simulink model "main"  (R2021a)
settings: Solver=ode45  StartTime=50  StopTime=60  RelTol=1e-3  EnableMultiTasking=on
undefined symbols (not defined in the file): Cadmium, Nickel
libraries: spsSeriesRLCBranchLib x4, spsGroundLib x3, spsControlledVoltageSourceLib x3, spsCurrentMeasurementLib x2, spsVoltageMeasurementLib x2, spspowerguiLib x2, spsBatteryLib x1, spsDiodeLib x1, spsMosfetLib x1, spsPWMGeneratorDCDCLib x1, spsUniversalBridgeLib x1
settings Model: Creator=Waqas vicky  LastModifiedBy=Le General
settings SolverCC: AlgebraicLoopSolver=TrustRegion
settings DataIOCC: LimitDataPoints=on  SaveFormat=Array  SignalLoggingSaveFormat=ModelDataLogs  ReturnWorkspaceOutputs=off
settings OptimizationCC: ExpressionDepthLimit=2147483647  LifeSpan=inf
settings DebuggingCC: UnderspecifiedInitializationDetection=Classic  MergeDetectMultiDrivingBlocksExec=none  SolverPrmCheckMsg=warning  FcnCallInpInsideContextMsg=warning  StateNameClashWarn=warning  SFUnexpectedBacktrackingDiag=warning  SFNoUnconditionalDefaultTransitionDiag=warning  SFExecutionAtInitializationDiag=none  SFMachineParentedDataDiag=warning  ArithmeticOperatorsInVariantConditions=warning
settings HardwareCC: ProdBitPerPointer=32  ProdBitPerSizeT=32  ProdBitPerPtrDiffT=32  ProdLargestAtomicFloat=None  ProdIntDivRoundTo=Undefined  ProdEndianess=Unspecified  ProdWordSize=32  ProdHWDeviceType=32-bit Generic
settings ModelReferenceCC: PropagateSignalLabelsOutOfModel=off
settings SFSimCC: SimUseLocalCustomCode=off  CustomCodeUndefinedFunction=UseInterfaceOnly
settings RTWCC: RTWUseLocalCustomCode=off
settings CodeAppCC: StateflowObjectComments=on
settings GRTTargetCC: TargetLangStandard=C89/C90 (ANSI)  CombineOutputUpdateFcns=off  GRTInterface=on
settings ConfigComp: CovMetricSettings=dw  CovSaveCumulativeToWorkspaceVar=on  CovSaveSingleToWorkspaceVar=on  CovExternalEMLEnable=off
settings SimscapeCC: SimscapeNormalizeSystem=off

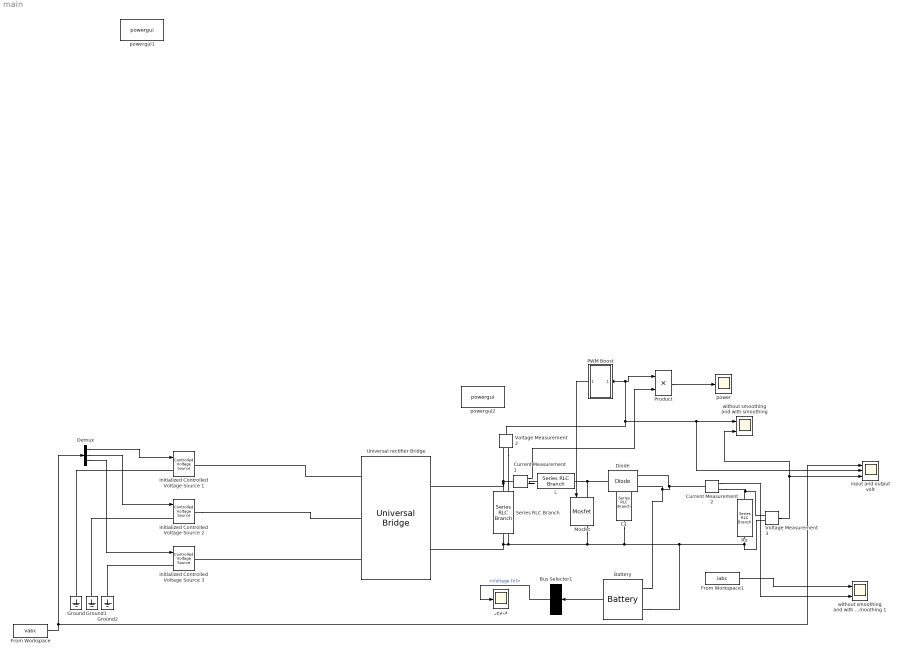
== system main ==
  Battery : spsBatteryLib/Battery  BatType=Nickel-Cadmium  ShowTempParam=off  ThermalPreset=no  ShowAgeParam=off  NomV=110  NomQ=5.4  SOC=100  Batt_Tr=30  PresetModel=off  MaxQ=6.1364  MinV=60  FullV=120  Dis_rate=1.08  R=0.088889  Normal_OP=5.1914  expZone="[120    1.50955]"  current=[6.5 13 32.5]  Units=Time  Tci=20  NomT=20  T2=-30  MaxQ2=4.8  FullV2=7.1  Normal_OP2=5.655  expZone2="[6.58           1]"  Rca=0.6  ti=2000  Dp=0  Neq0=0  Tsim=1e6  Ta1=25  Qeol=5.4*0.9  Reol=0.013333*1.2  Char_age=[2.3478, 3]  Dis_age=[2.3478, 10]  N1=1500  N2=10500  N3=1000  N4=1400  Ta2=45  N5=950
  Bus Selector1 : BusSelector  OutputSignals=Voltage (V)
  C1 : spsSeriesRLCBranchLib/Series RLC Branch  LConnTagsString=__new0  RConnTagsString=__new0  BranchType=C  Resistance=1  Inductance=1e-3  SetiL0=off  InitialCurrent=0  Capacitance=1  Setx0=off  InitialVoltage=0  Measurements=None
  Current Measurement1 : spsCurrentMeasurementLib/Current Measurement  PhasorSimulation=off  OutputType=Complex  PSBequivalent=0
  Current Measurement2 : spsCurrentMeasurementLib/Current Measurement  PhasorSimulation=off  OutputType=Complex  PSBequivalent=0
  Demux : Demux  Outputs=3
  Diode : spsDiodeLib/Diode  Ron=0.001  Lon=0  Vf=0.8  IC=0  UseSnubber=off  Rs=5000  Cs=250e-9  Measurements=on
  From Workspace : FromWorkspace  VariableName=vabc
  From Workspace1 : FromWorkspace  VariableName=iabc
  Ground : spsGroundLib/Ground  LConnTagsString=a
  Ground1 : spsGroundLib/Ground  LConnTagsString=a
  Ground2 : spsGroundLib/Ground  LConnTagsString=a
  Initialized Controlled Voltage Source 1 : spsControlledVoltageSourceLib/Controlled Voltage Source  Description=source block  Initialize=on  Source_Type=AC  Amplitude=120  Phase=0  Frequency=60  Measurements=None
      settings: AttributesFormatString=\n
  Initialized Controlled Voltage Source 2 : spsControlledVoltageSourceLib/Controlled Voltage Source  Description=source block  Initialize=on  Source_Type=AC  Amplitude=120  Phase=0  Frequency=60  Measurements=None
      settings: AttributesFormatString=\n
  Initialized Controlled Voltage Source 3 : spsControlledVoltageSourceLib/Controlled Voltage Source  Description=source block  Initialize=on  Source_Type=AC  Amplitude=120  Phase=0  Frequency=60  Measurements=None
      settings: AttributesFormatString=\n
  L : spsSeriesRLCBranchLib/Series RLC Branch  LConnTagsString=__new0  RConnTagsString=__new0  BranchType=L  Resistance=1  Inductance=6.5e-05  SetiL0=off  InitialCurrent=0  Capacitance=1e-6  Setx0=off  InitialVoltage=0  Measurements=None
  Mosfet : spsMosfetLib/Mosfet  Ron=0.1  Lon=0  Rd=0.01  Vfd=0  IC=0  Rs=1e5  Cs=inf  Measurements=on
  PWM Boost : Subsystem
  Product : Product
  Ro : spsSeriesRLCBranchLib/Series RLC Branch  LConnTagsString=__new0  RConnTagsString=__new0  BranchType=R  Resistance=15  Inductance=1e-3  SetiL0=off  InitialCurrent=0  Capacitance=1e-6  Setx0=off  InitialVoltage=0  Measurements=None
  Series RLC Branch : spsSeriesRLCBranchLib/Series RLC Branch  LConnTagsString=__new0  RConnTagsString=__new0  BranchType=C  Resistance=1  Inductance=1e-3  SetiL0=off  InitialCurrent=0  Capacitance=1e-06  Setx0=off  InitialVoltage=0  Measurements=None
  Universal rectifier Bridge : spsUniversalBridgeLib/Universal Bridge  Arms=3  SnubberResistance=10  SnubberCapacitance=inf  Device=Diodes  Ron=1e-3  Lon=0  ForwardVoltages="[  0  0  ]"  ForwardVoltage=0  GTOparameters=[ 10e-6 , 20e-6 ]  IGBTparameters=[ 1e-6 , 2e-6 ]  Measurements=None  Measurements_2=None  converterType=Rectifier
  Voltage Measurement2 : spsVoltageMeasurementLib/Voltage Measurement  PhasorSimulation=off  OutputType=Complex  PSBequivalent=0
  Voltage Measurement3 : spsVoltageMeasurementLib/Voltage Measurement  PhasorSimulation=off  OutputType=Complex  PSBequivalent=0
  input and output volt : Scope  NumInputPorts=3
  power : Scope
  powergui1 : spspowerguiLib/powergui  Priority=1  SimulationMode=Discrete  SampleTime=1e-6  frequency=60  Iterations=50  frequencyindice=0  Pbase=100e6  ErrMax=1e-4  UnitsV=kV  UnitsW=MW  buscounter=0  FunctionMessages=off  echomessages=off  EnableUseOfTLC=off  CurrentSourceSwitches=off  DisableSnubberDevices=off  DisableRonSwitches=off  DisableVfSwitches=off  DisplayEquations=off  AutomaticDiscreteSolvers=off  SolverType=Tustin/Backward Euler (TBE)  Interpol=off  ExternalGateDelay=off  methode=off  Ts=100  x0status=blocks  SPID=on  SwTol=0  HookPort=off  NonlinearTolerance=1e-4  nMaxIteration=100  ContinueOnMaxIteration=off  RestoreLinks=warning  ResistiveCurrentMeasurement=off  Frange=[0:2:500]  Ylog=off  Xlog=on  ShowGrid=off  save=off  variable=ZData  structure=0  ZoomFFT=off  StartTime=0.0  cycles=1  DisplayStyle=1  fundamental=60  FreqAxis=off  MaxFrequency=1000  frequencyindicesteady=1  RmsSteady=1  display=off
  powergui2 : spspowerguiLib/powergui  Priority=1  SimulationMode=Discrete  SampleTime=1e-6  frequency=60  Iterations=50  frequencyindice=0  Pbase=100e6  ErrMax=1e-4  UnitsV=kV  UnitsW=MW  buscounter=0  FunctionMessages=off  echomessages=off  EnableUseOfTLC=off  CurrentSourceSwitches=off  DisableSnubberDevices=off  DisableRonSwitches=off  DisableVfSwitches=off  DisplayEquations=off  AutomaticDiscreteSolvers=off  SolverType=Tustin/Backward Euler (TBE)  Interpol=off  ExternalGateDelay=off  methode=off  Ts=100  x0status=blocks  SPID=on  SwTol=0  HookPort=off  NonlinearTolerance=1e-4  nMaxIteration=100  ContinueOnMaxIteration=off  RestoreLinks=warning  ResistiveCurrentMeasurement=off  Frange=[0:2:500]  Ylog=off  Xlog=on  ShowGrid=off  save=off  variable=ZData  structure=0  ZoomFFT=off  StartTime=0.0  cycles=1  DisplayStyle=1  fundamental=60  FreqAxis=off  MaxFrequency=1000  frequencyindicesteady=1  RmsSteady=1  display=off
  "without smoothing and with smoothing " : Scope  NumInputPorts=2
  without smoothing and with smoothing 1 : Scope  NumInputPorts=2
  رخمف : Scope
  wires:
  From Workspace/1 -> input and output volt/1, Demux/1
  Demux/1 -> Initialized Controlled Voltage Source 1/1
  Demux/3 -> Initialized Controlled Voltage Source 3/1
  Demux/2 -> Initialized Controlled Voltage Source 2/1
  Voltage Measurement3/1 -> "without smoothing and with smoothing "/2, input and output volt/3
  PWM Boost/1(Out1) -> Mosfet/1
  Battery/1 -> Bus Selector1/1
  Current Measurement1/1 -> Product/2
  Voltage Measurement2/1 -> input and output volt/2, "without smoothing and with smoothing "/1, Product/1, PWM Boost/1(In1)
  Product/1 -> power/1
  Bus Selector1/1 -> رخمف/1  "<Voltage (V)>"
  From Workspace1/1 -> without smoothing and with smoothing 1/1
  Current Measurement2/1 -> without smoothing and with smoothing 1/2
  connections:
  Ground2/LConn1 -- Initialized Controlled Voltage Source 3/LConn1
  Ground1/LConn1 -- Initialized Controlled Voltage Source 2/LConn1
  Ground/LConn1 -- Initialized Controlled Voltage Source 1/LConn1
  Current Measurement1/LConn1 -- Series RLC Branch/RConn1 -- Universal rectifier Bridge/RConn1 -- Voltage Measurement2/LConn1
  L/RConn1 -- Mosfet/LConn1 -- Diode/LConn1
  Series RLC Branch/LConn1 -- Battery/LConn2 -- Voltage Measurement3/LConn2 -- Ro/RConn1 -- C1/RConn1 -- Mosfet/RConn1 -- Voltage Measurement2/LConn2 -- Universal rectifier Bridge/RConn2
  Voltage Measurement3/LConn1 -- Current Measurement2/RConn1 -- Ro/LConn1
  Current Measurement1/RConn1 -- L/LConn1
  Universal rectifier Bridge/LConn1 -- Initialized Controlled Voltage Source 1/RConn1
  Initialized Controlled Voltage Source 2/RConn1 -- Universal rectifier Bridge/LConn2
  Universal rectifier Bridge/LConn3 -- Initialized Controlled Voltage Source 3/RConn1
  Battery/LConn1 -- Current Measurement2/LConn1 -- C1/LConn1 -- Diode/RConn1

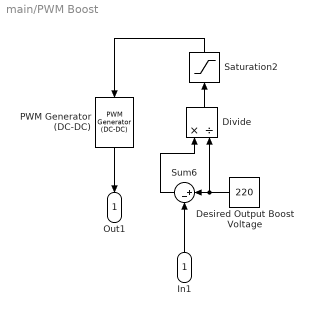
== system main/PWM Boost ==
  In1 : Inport
  Desired Output Boost Voltage : Constant  Value=220
  Divide : Product  Inputs=*/
  PWM Generator (DC-DC) : spsPWMGeneratorDCDCLib/PWM Generator (DC-DC)  Fsw=25000  Ts=0
  Saturation2 : Saturate  UpperLimit=0.95  LowerLimit=0.1
  Sum6 : Sum  Inputs=|+-
  Out1 : Outport  VectorParamsAs1DForOutWhenUnconnected=off
  wires:
  Divide/1 -> Saturation2/1
  Desired Output Boost Voltage/1 -> Sum6/1, Divide/2
  PWM Generator (DC-DC)/1 -> Out1/1
  Sum6/1 -> Divide/1
  Saturation2/1 -> PWM Generator (DC-DC)/1
  In1/1 -> Sum6/2
